simulink library "IOBlock_Library_TTC580"  (R2021a)
settings: Solver=ode45  StartTime=0.0  StopTime=10.0  RelTol=1e-3
PreLoadFcn:
  | addpath(genpath(fileparts(which('IOBlock_Library_TTC580'))));
  | %addpath(genpath(fileparts(which('IOBlock_Library_TTC580.mdl'))))
  | try
  | addpath(genpath([fileparts(which('IOBlock_Library_TTC580')),'\..\DBC_Importer']));
  | addpath(genpath([fileparts(which('IOBlock_Library_TTC580')),'\..\EEPROM_Importer']));
  | addpath(genpath([fileparts(which('IOBlock_Library_TTC580')),'\..\UserDoc']));
  | catch
  | warning('IOBlock_Library_TTC580: add path to DBC_Importer and EEPROM_Importer manually');
  | end
  | try
  | if exist('..\CustomPackage\scripts\OpenAllPackages.m','file')
  |      run('..\CustomPackage\scripts\OpenAllPackages.m'); %always available, ggf. empty
  | end
  | catch
  | warning('A problem occurred opening automatically the CustomPackage. Please open libraries manually');
  | end
  | try
  | set_param(0,'EditorSmartEditingHotParam','off');
  | catch
  | warning('Simlink preferences for ''Edit key parameter when adding new blocks'' needs to be unchecked manually');
  | end
undefined symbols (not defined in the file or in its folder): ADC_Absolute_10V, ADC_Absolute_32V, ADC_Absolute_5V, ADC_BoardTemp, ADC_ChannelInit, ADC_Current, ADC_Get, ADC_K15_, ADC_Ratiometric_10V, ADC_Ratiometric_5V, ADC_Resistive, ADC_SensorSupply, ADC_UBAT, bit_packing, bit_unpacking, CAN_ConfigMsg, compare2error, compare2FET_PROT_REENABLE, crc32_calc_intern, CRC32_EEPROM_Read, CRC32_EEPROM_Write, DIAG_EnterSafestate, DIAG_Status, DIAG_Status_internal, EEPROM_Mirror, EEPROM_Read, EEPROM_Read_OffsetIn, EEPROM_Read_Raw, EEPROM_Write, EEPROM_Write_OffsetIn, EEPROM_Write_Raw, EnterSafestate, FPU_Handler, Get_DI, Get_DI_VarThreshold, Get_K15_, Get_Pulse_Freq_Curr, Get_Pulse_Freq_Volt, Get_WakeUp, GetDateAndTime, IO_ADC_ResetProtection, IO_Blk_Lib_TTC500, IO_CAN_ReadMsg, IO_CAN_WriteMsg, IO_DI_Get, IO_DI_Init, IO_DI_Init_Var, IO_DO_GetCur, IO_DO_GetVoltage, IO_DO_Init, IO_DO_ResetProtection, IO_DO_Set, IO_Driver_GetSerialNumber, IO_Driver_GetVersionOfDriver, IO_Driver_GetVersionOfFPGA, IO_EEPROM_GetStatus, IO_EEPROM_Init, IO_EEPROM_Read_raw, IO_EEPROM_Write, IO_EEPROM_Write_OffsetIn ... (+73)
libraries: simulink x43
(part 17 of 18)

== system IOBlock_Library_TTC580/EEPROM Blocks TTC580 IOlib/EEPROM_Write/IO_EEPROM_Write ==
  EC_Write_Mirror : Inport
  GetStatus : Inport  Port=2
  IO_EEPROM_Write_s : S-Function  FunctionName=IO_EEPROM_Write_s  Parameters=SampleTime,offset,length  SFunctionDeploymentMode=off  EnableBusSupport=off
  ErrorCode : Outport  VectorParamsAs1DForOutWhenUnconnected=off
  wires:
  IO_EEPROM_Write_s/1 -> ErrorCode/1
  GetStatus/1 -> IO_EEPROM_Write_s/2
  EC_Write_Mirror/1 -> IO_EEPROM_Write_s/1

== system IOBlock_Library_TTC580/EEPROM Blocks TTC580 IOlib/EEPROM_Write/Write_Mirror ==
  b_trigger : Inport
  data : Inport  Port=2
  Write_Mirror_s : S-Function  FunctionName=Write_Mirror_s  Parameters=SampleTime,offset,length  SFunctionDeploymentMode=off  EnableBusSupport=off
  ErrorCode_EEPROM_mirror : Outport  VectorParamsAs1DForOutWhenUnconnected=off
  wires:
  Write_Mirror_s/1 -> ErrorCode_EEPROM_mirror/1
  data/1 -> Write_Mirror_s/2
  b_trigger/1 -> Write_Mirror_s/1

== system IOBlock_Library_TTC580/EEPROM Blocks TTC580 IOlib/EEPROM_Write_OffsetIn/EEPROM_Mirror ==
  EC_EEPROM_Init : Inport
  EEPROM_Mirror_s : S-Function  FunctionName=EEPROM_Mirror_s  Parameters=SampleTime,offset,length  SFunctionDeploymentMode=off  EnableBusSupport=off
  Terminator : Terminator
  wires:
  EEPROM_Mirror_s/1 -> Terminator/1
  EC_EEPROM_Init/1 -> EEPROM_Mirror_s/1

== system IOBlock_Library_TTC580/EEPROM Blocks TTC580 IOlib/EEPROM_Write_OffsetIn/IO_EEPROM_GetStatus ==
  IO_EEPROM_GetStatus_s : S-Function  FunctionName=IO_EEPROM_GetStatus_s  Parameters=SampleTime  SFunctionDeploymentMode=off  EnableBusSupport=off
  ErrorCode : Outport  VectorParamsAs1DForOutWhenUnconnected=off
  wires:
  IO_EEPROM_GetStatus_s/1 -> ErrorCode/1

== system IOBlock_Library_TTC580/EEPROM Blocks TTC580 IOlib/EEPROM_Write_OffsetIn/IO_EEPROM_GetStatus1 ==
  IO_EEPROM_GetStatus_s : S-Function  FunctionName=IO_EEPROM_GetStatus_s  Parameters=SampleTime  SFunctionDeploymentMode=off  EnableBusSupport=off
  ErrorCode : Outport  VectorParamsAs1DForOutWhenUnconnected=off
  wires:
  IO_EEPROM_GetStatus_s/1 -> ErrorCode/1

== system IOBlock_Library_TTC580/EEPROM Blocks TTC580 IOlib/EEPROM_Write_OffsetIn/IO_EEPROM_Init ==
  IO_EEPROM_Init_s : S-Function  FunctionName=IO_EEPROM_Init_s  Parameters=SampleTime  SFunctionDeploymentMode=off  EnableBusSupport=off
  ErrorCode : Outport  VectorParamsAs1DForOutWhenUnconnected=off
  wires:
  IO_EEPROM_Init_s/1 -> ErrorCode/1

== system IOBlock_Library_TTC580/EEPROM Blocks TTC580 IOlib/EEPROM_Write_OffsetIn/IO_EEPROM_Write_OffsetIn ==
  offset : Inport
  EC_Write_Mirror : Inport  Port=2
  GetStatus : Inport  Port=3
  IO_EEPROM_Write_OffsetIn_s : S-Function  FunctionName=IO_EEPROM_Write_OffsetIn_s  Parameters=SampleTime,length  SFunctionDeploymentMode=off  EnableBusSupport=off
  ErrorCode : Outport  VectorParamsAs1DForOutWhenUnconnected=off
  wires:
  IO_EEPROM_Write_OffsetIn_s/1 -> ErrorCode/1
  GetStatus/1 -> IO_EEPROM_Write_OffsetIn_s/3
  EC_Write_Mirror/1 -> IO_EEPROM_Write_OffsetIn_s/2
  offset/1 -> IO_EEPROM_Write_OffsetIn_s/1

== system IOBlock_Library_TTC580/EEPROM Blocks TTC580 IOlib/EEPROM_Write_OffsetIn/Write_Mirror_OffsetIn ==
  offset : Inport
  b_trigger : Inport  Port=2
  data : Inport  Port=3
  Write_Mirror_OffsetIn_s : S-Function  FunctionName=Write_Mirror_OffsetIn_s  Parameters=SampleTime,length  SFunctionDeploymentMode=off  EnableBusSupport=off
  ErrorCode_EEPROM_mirror : Outport  VectorParamsAs1DForOutWhenUnconnected=off
  wires:
  Write_Mirror_OffsetIn_s/1 -> ErrorCode_EEPROM_mirror/1
  data/1 -> Write_Mirror_OffsetIn_s/3
  b_trigger/1 -> Write_Mirror_OffsetIn_s/2
  offset/1 -> Write_Mirror_OffsetIn_s/1

== system IOBlock_Library_TTC580/EEPROM Blocks TTC580 IOlib/EEPROM_Write_Raw/IO_EEPROM_Init ==
  IO_EEPROM_Init_s : S-Function  FunctionName=IO_EEPROM_Init_s  Parameters=SampleTime  SFunctionDeploymentMode=off  EnableBusSupport=off
  ErrorCode : Outport  VectorParamsAs1DForOutWhenUnconnected=off
  wires:
  IO_EEPROM_Init_s/1 -> ErrorCode/1

== system IOBlock_Library_TTC580/EEPROM Blocks TTC580 IOlib/EEPROM_Write_Raw/IO_EEPROM_Write_raw ==
  data : Inport
  IO_EEPROM_Write_raw_s : S-Function  FunctionName=IO_EEPROM_Write_raw_s  Parameters=SampleTime,offset,length  SFunctionDeploymentMode=off  EnableBusSupport=off
  ErrorCode : Outport  VectorParamsAs1DForOutWhenUnconnected=off
  wires:
  IO_EEPROM_Write_raw_s/1 -> ErrorCode/1
  data/1 -> IO_EEPROM_Write_raw_s/1

== system IOBlock_Library_TTC580/LIN TTC580 IOlib/IO_LIN_Init/IO_LIN_Init ==
  baudrate : Inport
  checksum_type : Inport  Port=2
  IO_LIN_Init_s : S-Function  FunctionName=IO_LIN_Init_s  Parameters=SampleTime  SFunctionDeploymentMode=off  EnableBusSupport=off
  ErrorCode : Outport  VectorParamsAs1DForOutWhenUnconnected=off
  wires:
  IO_LIN_Init_s/1 -> ErrorCode/1
  checksum_type/1 -> IO_LIN_Init_s/2
  baudrate/1 -> IO_LIN_Init_s/1

== system IOBlock_Library_TTC580/LIN TTC580 IOlib/LIN_Read/LIN_Read_intern ==
  frame_id : Inport
  frame_length : Inport  Port=2
  b_reqst : Inport  Port=3
  LIN_Read_intern_s : S-Function  FunctionName=LIN_Read_intern_s  Parameters=SampleTime  SFunctionDeploymentMode=off  EnableBusSupport=off
  ErrorCode : Outport  VectorParamsAs1DForOutWhenUnconnected=off
  frame_data : Outport  Port=2  VectorParamsAs1DForOutWhenUnconnected=off
  wires:
  LIN_Read_intern_s/2 -> frame_data/1
  LIN_Read_intern_s/1 -> ErrorCode/1
  b_reqst/1 -> LIN_Read_intern_s/3
  frame_length/1 -> LIN_Read_intern_s/2
  frame_id/1 -> LIN_Read_intern_s/1

== system IOBlock_Library_TTC580/LIN TTC580 IOlib/LIN_Write/IO_LIN_Write ==
  frame_id : Inport
  frame_length : Inport  Port=2
  frame_data : Inport  Port=3
  Enable : EnablePort
  IO_LIN_Write_s : S-Function  FunctionName=IO_LIN_Write_s  Parameters=SampleTime  SFunctionDeploymentMode=off  EnableBusSupport=off
  ErrorCode : Outport  VectorParamsAs1DForOutWhenUnconnected=off
  wires:
  IO_LIN_Write_s/1 -> ErrorCode/1
  frame_data/1 -> IO_LIN_Write_s/3
  frame_length/1 -> IO_LIN_Write_s/2
  frame_id/1 -> IO_LIN_Write_s/1

== system IOBlock_Library_TTC580/PVG and VOUT TTC580 IOlib/Set_PVG_Simple/IO_PVG_Init ==
  IO_PVG_Init_s : S-Function  FunctionName=IO_PVG_Init_s  Parameters=SampleTime,pvg_channel,init_output_value  SFunctionDeploymentMode=off  EnableBusSupport=off
  ErrorCode : Outport  VectorParamsAs1DForOutWhenUnconnected=off
  wires:
  IO_PVG_Init_s/1 -> ErrorCode/1

== system IOBlock_Library_TTC580/PVG and VOUT TTC580 IOlib/Set_PVG_Simple/IO_PVG_ResetProtection ==
  Trigger : TriggerPort  VariantControl=(inherit)
  IO_PVG_ResetProtection_s : S-Function  FunctionName=IO_PVG_ResetProtection_s  Parameters=SampleTime,pvg_channel  SFunctionDeploymentMode=off  EnableBusSupport=off
  ErrorCode : Outport  VectorParamsAs1DForOutWhenUnconnected=off
  reset_cnt : Outport  Port=2  VectorParamsAs1DForOutWhenUnconnected=off
  wires:
  IO_PVG_ResetProtection_s/2 -> reset_cnt/1
  IO_PVG_ResetProtection_s/1 -> ErrorCode/1

== system IOBlock_Library_TTC580/PVG and VOUT TTC580 IOlib/Set_PVG_Simple/IO_PVG_SetOutput ==
  output_value : Inport
  IO_PVG_SetOutput_s : S-Function  FunctionName=IO_PVG_SetOutput_s  Parameters=SampleTime,pvg_channel  SFunctionDeploymentMode=off  EnableBusSupport=off
  ErrorCode : Outport  VectorParamsAs1DForOutWhenUnconnected=off
  wires:
  IO_PVG_SetOutput_s/1 -> ErrorCode/1
  output_value/1 -> IO_PVG_SetOutput_s/1

== system IOBlock_Library_TTC580/PVG and VOUT TTC580 IOlib/Set_PVG_Simple/compare2FET_PROT_REENABLE ==
  Errorcode : Inport  OutDataTypeStr=uint16
  compare2error_s : S-Function  FunctionName=compare2error_s  Parameters=SampleTime,define  SFunctionDeploymentMode=off  EnableBusSupport=off
  b_compare : Outport  VectorParamsAs1DForOutWhenUnconnected=off
  wires:
  compare2error_s/1 -> b_compare/1
  Errorcode/1 -> compare2error_s/1

== system IOBlock_Library_TTC580/PVG and VOUT TTC580 IOlib/Set_PVG_VoltFb/IO_PVG_GetVoltage ==
  IO_PVG_GetVoltage_s : S-Function  FunctionName=IO_PVG_GetVoltage_s  Parameters=SampleTime,pvg_channel  SFunctionDeploymentMode=off  EnableBusSupport=off
  ErrorCode : Outport  VectorParamsAs1DForOutWhenUnconnected=off
  voltage : Outport  Port=2  VectorParamsAs1DForOutWhenUnconnected=off
  fresh : Outport  Port=3  VectorParamsAs1DForOutWhenUnconnected=off
  wires:
  IO_PVG_GetVoltage_s/3 -> fresh/1
  IO_PVG_GetVoltage_s/2 -> voltage/1
  IO_PVG_GetVoltage_s/1 -> ErrorCode/1

== system IOBlock_Library_TTC580/PVG and VOUT TTC580 IOlib/Set_PVG_VoltFb/IO_PVG_Init ==
  IO_PVG_Init_s : S-Function  FunctionName=IO_PVG_Init_s  Parameters=SampleTime,pvg_channel,init_output_value  SFunctionDeploymentMode=off  EnableBusSupport=off
  ErrorCode : Outport  VectorParamsAs1DForOutWhenUnconnected=off
  wires:
  IO_PVG_Init_s/1 -> ErrorCode/1

== system IOBlock_Library_TTC580/PVG and VOUT TTC580 IOlib/Set_PVG_VoltFb/IO_PVG_ResetProtection ==
  Trigger : TriggerPort  VariantControl=(inherit)
  IO_PVG_ResetProtection_s : S-Function  FunctionName=IO_PVG_ResetProtection_s  Parameters=SampleTime,pvg_channel  SFunctionDeploymentMode=off  EnableBusSupport=off
  ErrorCode : Outport  VectorParamsAs1DForOutWhenUnconnected=off
  reset_cnt : Outport  Port=2  VectorParamsAs1DForOutWhenUnconnected=off
  wires:
  IO_PVG_ResetProtection_s/1 -> ErrorCode/1
  IO_PVG_ResetProtection_s/2 -> reset_cnt/1

== system IOBlock_Library_TTC580/PVG and VOUT TTC580 IOlib/Set_PVG_VoltFb/IO_PVG_SetOutput ==
  output_value : Inport
  IO_PVG_SetOutput_s : S-Function  FunctionName=IO_PVG_SetOutput_s  Parameters=SampleTime,pvg_channel  SFunctionDeploymentMode=off  EnableBusSupport=off
  ErrorCode : Outport  VectorParamsAs1DForOutWhenUnconnected=off
  wires:
  output_value/1 -> IO_PVG_SetOutput_s/1
  IO_PVG_SetOutput_s/1 -> ErrorCode/1

== system IOBlock_Library_TTC580/PVG and VOUT TTC580 IOlib/Set_PVG_VoltFb/compare2FET_PROT_REENABLE ==
  Errorcode : Inport  OutDataTypeStr=uint16
  compare2error_s : S-Function  FunctionName=compare2error_s  Parameters=SampleTime,define  SFunctionDeploymentMode=off  EnableBusSupport=off
  b_compare : Outport  VectorParamsAs1DForOutWhenUnconnected=off
  wires:
  Errorcode/1 -> compare2error_s/1
  compare2error_s/1 -> b_compare/1

== system IOBlock_Library_TTC580/PVG and VOUT TTC580 IOlib/Set_VOUT_Simple/IO_VOUT_Init ==
  IO_VOUT_Init_s : S-Function  FunctionName=IO_VOUT_Init_s  Parameters=SampleTime,vout_channel  SFunctionDeploymentMode=off  EnableBusSupport=off
  ErrorCode : Outport  VectorParamsAs1DForOutWhenUnconnected=off
  wires:
  IO_VOUT_Init_s/1 -> ErrorCode/1

== system IOBlock_Library_TTC580/PVG and VOUT TTC580 IOlib/Set_VOUT_Simple/IO_VOUT_ResetProtection ==
  Trigger : TriggerPort  VariantControl=(inherit)
  IO_VOUT_ResetProtection_s : S-Function  FunctionName=IO_VOUT_ResetProtection_s  Parameters=SampleTime,vout_channel  SFunctionDeploymentMode=off  EnableBusSupport=off
  ErrorCode : Outport  VectorParamsAs1DForOutWhenUnconnected=off
  reset_cnt : Outport  Port=2  VectorParamsAs1DForOutWhenUnconnected=off
  wires:
  IO_VOUT_ResetProtection_s/2 -> reset_cnt/1
  IO_VOUT_ResetProtection_s/1 -> ErrorCode/1

== system IOBlock_Library_TTC580/PVG and VOUT TTC580 IOlib/Set_VOUT_Simple/IO_VOUT_SetVoltage ==
  output_voltage : Inport
  IO_VOUT_SetVoltage_s : S-Function  FunctionName=IO_VOUT_SetVoltage_s  Parameters=SampleTime,vout_channel  SFunctionDeploymentMode=off  EnableBusSupport=off
  ErrorCode : Outport  VectorParamsAs1DForOutWhenUnconnected=off
  wires:
  IO_VOUT_SetVoltage_s/1 -> ErrorCode/1
  output_voltage/1 -> IO_VOUT_SetVoltage_s/1

== system IOBlock_Library_TTC580/PVG and VOUT TTC580 IOlib/Set_VOUT_Simple/compare2FET_PROT_REENABLE ==
  Errorcode : Inport  OutDataTypeStr=uint16
  compare2error_s : S-Function  FunctionName=compare2error_s  Parameters=SampleTime,define  SFunctionDeploymentMode=off  EnableBusSupport=off
  b_compare : Outport  VectorParamsAs1DForOutWhenUnconnected=off
  wires:
  Errorcode/1 -> compare2error_s/1
  compare2error_s/1 -> b_compare/1

== system IOBlock_Library_TTC580/PVG and VOUT TTC580 IOlib/Set_VOUT_VoltFb/IO_VOUT_GetVoltage ==
  IO_VOUT_GetVoltage_s : S-Function  FunctionName=IO_VOUT_GetVoltage_s  Parameters=SampleTime,vout_channel  SFunctionDeploymentMode=off  EnableBusSupport=off
  ErrorCode : Outport  VectorParamsAs1DForOutWhenUnconnected=off
  voltage : Outport  Port=2  VectorParamsAs1DForOutWhenUnconnected=off
  fresh : Outport  Port=3  VectorParamsAs1DForOutWhenUnconnected=off
  wires:
  IO_VOUT_GetVoltage_s/3 -> fresh/1
  IO_VOUT_GetVoltage_s/2 -> voltage/1
  IO_VOUT_GetVoltage_s/1 -> ErrorCode/1

== system IOBlock_Library_TTC580/PVG and VOUT TTC580 IOlib/Set_VOUT_VoltFb/IO_VOUT_Init ==
  IO_VOUT_Init_s : S-Function  FunctionName=IO_VOUT_Init_s  Parameters=SampleTime,vout_channel  SFunctionDeploymentMode=off  EnableBusSupport=off
  ErrorCode : Outport  VectorParamsAs1DForOutWhenUnconnected=off
  wires:
  IO_VOUT_Init_s/1 -> ErrorCode/1

== system IOBlock_Library_TTC580/PVG and VOUT TTC580 IOlib/Set_VOUT_VoltFb/IO_VOUT_ResetProtection ==
  Trigger : TriggerPort  VariantControl=(inherit)
  IO_VOUT_ResetProtection_s : S-Function  FunctionName=IO_VOUT_ResetProtection_s  Parameters=SampleTime,vout_channel  SFunctionDeploymentMode=off  EnableBusSupport=off
  ErrorCode : Outport  VectorParamsAs1DForOutWhenUnconnected=off
  reset_cnt : Outport  Port=2  VectorParamsAs1DForOutWhenUnconnected=off
  wires:
  IO_VOUT_ResetProtection_s/1 -> ErrorCode/1
  IO_VOUT_ResetProtection_s/2 -> reset_cnt/1

== system IOBlock_Library_TTC580/PVG and VOUT TTC580 IOlib/Set_VOUT_VoltFb/IO_VOUT_SetVoltage ==
  output_voltage : Inport
  IO_VOUT_SetVoltage_s : S-Function  FunctionName=IO_VOUT_SetVoltage_s  Parameters=SampleTime,vout_channel  SFunctionDeploymentMode=off  EnableBusSupport=off
  ErrorCode : Outport  VectorParamsAs1DForOutWhenUnconnected=off
  wires:
  output_voltage/1 -> IO_VOUT_SetVoltage_s/1
  IO_VOUT_SetVoltage_s/1 -> ErrorCode/1

== system IOBlock_Library_TTC580/PVG and VOUT TTC580 IOlib/Set_VOUT_VoltFb/compare2FET_PROT_REENABLE ==
  Errorcode : Inport  OutDataTypeStr=uint16
  compare2error_s : S-Function  FunctionName=compare2error_s  Parameters=SampleTime,define  SFunctionDeploymentMode=off  EnableBusSupport=off
  b_compare : Outport  VectorParamsAs1DForOutWhenUnconnected=off
  wires:
  compare2error_s/1 -> b_compare/1
  Errorcode/1 -> compare2error_s/1

== system IOBlock_Library_TTC580/PWD Blocks TTC580 IOlib/Get_Pulse_Freq_Curr/IO_PWD_ComplexGet ==
  IO_PWD_ComplexGet_s : S-Function  FunctionName=IO_PWD_ComplexGet_s  Parameters=SampleTime,timer_channel,pin_value,pulse_samples  SFunctionDeploymentMode=off  EnableBusSupport=off
  ErrorCode : Outport  VectorParamsAs1DForOutWhenUnconnected=off
  frequency : Outport  Port=2  VectorParamsAs1DForOutWhenUnconnected=off
  pulse_width : Outport  Port=3  VectorParamsAs1DForOutWhenUnconnected=off
  wires:
  IO_PWD_ComplexGet_s/3 -> pulse_width/1
  IO_PWD_ComplexGet_s/2 -> frequency/1
  IO_PWD_ComplexGet_s/1 -> ErrorCode/1

== system IOBlock_Library_TTC580/PWD Blocks TTC580 IOlib/Get_Pulse_Freq_Curr/IO_PWD_ResetProtection ==
  Trigger : TriggerPort  VariantControl=(inherit)
  IO_PWD_ResetProtection_s : S-Function  FunctionName=IO_PWD_ResetProtection_s  Parameters=SampleTime,pwd_channel  SFunctionDeploymentMode=off  EnableBusSupport=off
  ErrorCode : Outport  VectorParamsAs1DForOutWhenUnconnected=off
  reset_cnt : Outport  Port=2  VectorParamsAs1DForOutWhenUnconnected=off
  wires:
  IO_PWD_ResetProtection_s/2 -> reset_cnt/1
  IO_PWD_ResetProtection_s/1 -> ErrorCode/1

== system IOBlock_Library_TTC580/PWD Blocks TTC580 IOlib/Get_Pulse_Freq_Curr/PWD_ComplexInit ==
  PWD_ComplexInit_s : S-Function  FunctionName=PWD_ComplexInit_s  Parameters=SampleTime,timer_channel,pulse_mode,freq_mode,capture_count,pupd,safety_conf  SFunctionDeploymentMode=off  EnableBusSupport=off
  ErrorCode : Outport  VectorParamsAs1DForOutWhenUnconnected=off
  wires:
  PWD_ComplexInit_s/1 -> ErrorCode/1

== system IOBlock_Library_TTC580/PWD Blocks TTC580 IOlib/Get_Pulse_Freq_Curr/compare2FET_PROT_REENABLE ==
  Errorcode : Inport  OutDataTypeStr=uint16
  compare2error_s : S-Function  FunctionName=compare2error_s  Parameters=SampleTime,define  SFunctionDeploymentMode=off  EnableBusSupport=off
  b_compare : Outport  VectorParamsAs1DForOutWhenUnconnected=off
  wires:
  compare2error_s/1 -> b_compare/1
  Errorcode/1 -> compare2error_s/1

== system IOBlock_Library_TTC580/PWD Blocks TTC580 IOlib/Get_Pulse_Freq_Volt/IO_PWD_ComplexGet ==
  IO_PWD_ComplexGet_s : S-Function  FunctionName=IO_PWD_ComplexGet_s  Parameters=SampleTime,timer_channel,pin_value,pulse_samples  SFunctionDeploymentMode=off  EnableBusSupport=off
  ErrorCode : Outport  VectorParamsAs1DForOutWhenUnconnected=off
  frequency : Outport  Port=2  VectorParamsAs1DForOutWhenUnconnected=off
  pulse_width : Outport  Port=3  VectorParamsAs1DForOutWhenUnconnected=off
  wires:
  IO_PWD_ComplexGet_s/1 -> ErrorCode/1
  IO_PWD_ComplexGet_s/2 -> frequency/1
  IO_PWD_ComplexGet_s/3 -> pulse_width/1

== system IOBlock_Library_TTC580/PWD Blocks TTC580 IOlib/Get_Pulse_Freq_Volt/PWD_ComplexInit ==
  PWD_ComplexInit_s : S-Function  FunctionName=PWD_ComplexInit_s  Parameters=SampleTime,timer_channel,pulse_mode,freq_mode,capture_count,pupd,safety_conf  SFunctionDeploymentMode=off  EnableBusSupport=off
  ErrorCode : Outport  VectorParamsAs1DForOutWhenUnconnected=off
  wires:
  PWD_ComplexInit_s/1 -> ErrorCode/1

== system IOBlock_Library_TTC580/PWD Blocks TTC580 IOlib/PWD_Inc/PWD_IncGet ==
  PWD_IncGet_s : S-Function  FunctionName=PWD_IncGet_s  Parameters=SampleTime,inc_channel,pin_value_0,pin_value_1  SFunctionDeploymentMode=off  EnableBusSupport=off
  ErrorCode : Outport  VectorParamsAs1DForOutWhenUnconnected=off
  count : Outport  Port=2  VectorParamsAs1DForOutWhenUnconnected=off
  wires:
  PWD_IncGet_s/1 -> ErrorCode/1
  PWD_IncGet_s/2 -> count/1

== system IOBlock_Library_TTC580/PWD Blocks TTC580 IOlib/PWD_Inc/PWD_IncInit ==
  PWD_IncInit_s : S-Function  FunctionName=PWD_IncInit_s  Parameters=SampleTime,inc_channel,mode,count_init,pupd,safety_conf  SFunctionDeploymentMode=off  EnableBusSupport=off
  ErrorCode : Outport  VectorParamsAs1DForOutWhenUnconnected=off
  wires:
  PWD_IncInit_s/1 -> ErrorCode/1

== system IOBlock_Library_TTC580/PWD Blocks TTC580 IOlib/PWD_IncReset/PWD_IncSet_Internal ==
  count : Inport
  Trigger : TriggerPort  VariantControl=(inherit)
  PWD_IncSet_Internal_s : S-Function  FunctionName=PWD_IncSet_Internal_s  Parameters=SampleTime,inc_channel  SFunctionDeploymentMode=off  EnableBusSupport=off
  ErrorCode : Outport  VectorParamsAs1DForOutWhenUnconnected=off
  wires:
  count/1 -> PWD_IncSet_Internal_s/1
  PWD_IncSet_Internal_s/1 -> ErrorCode/1

== system IOBlock_Library_TTC580/PWM Blocks TTC580 IOlib/Set_PWM_CurrFb/IO_PWM_GetCur ==
  IO_PWM_GetCur_s : S-Function  FunctionName=IO_PWM_GetCur_s  Parameters=SampleTime,pwm_channel  SFunctionDeploymentMode=off  EnableBusSupport=off
  ErrorCode : Outport  VectorParamsAs1DForOutWhenUnconnected=off
  current : Outport  Port=2  VectorParamsAs1DForOutWhenUnconnected=off
  fresh : Outport  Port=3  VectorParamsAs1DForOutWhenUnconnected=off
  wires:
  IO_PWM_GetCur_s/1 -> ErrorCode/1
  IO_PWM_GetCur_s/2 -> current/1
  IO_PWM_GetCur_s/3 -> fresh/1

== system IOBlock_Library_TTC580/PWM Blocks TTC580 IOlib/Set_PWM_CurrFb/IO_PWM_Init ==
  IO_PWM_Init_s : S-Function  FunctionName=IO_PWM_Init_s  Parameters=SampleTime,pwm_channel,frequency,polarity,diag_margin,safety_conf  SFunctionDeploymentMode=off  EnableBusSupport=off
  ErrorCode : Outport  VectorParamsAs1DForOutWhenUnconnected=off
  wires:
  IO_PWM_Init_s/1 -> ErrorCode/1

== system IOBlock_Library_TTC580/PWM Blocks TTC580 IOlib/Set_PWM_CurrFb/IO_PWM_ResetProtection ==
  Trigger : TriggerPort  VariantControl=(inherit)
  IO_PWM_ResetProtection_s : S-Function  FunctionName=IO_PWM_ResetProtection_s  Parameters=SampleTime,pwm_channel  SFunctionDeploymentMode=off  EnableBusSupport=off
  ErrorCode : Outport  VectorParamsAs1DForOutWhenUnconnected=off
  reset_cnt : Outport  Port=2  VectorParamsAs1DForOutWhenUnconnected=off
  wires:
  IO_PWM_ResetProtection_s/1 -> ErrorCode/1
  IO_PWM_ResetProtection_s/2 -> reset_cnt/1

== system IOBlock_Library_TTC580/PWM Blocks TTC580 IOlib/Set_PWM_CurrFb/PWM_SetDuty_Simple ==
  duty_cycle : Inport
  PWM_SetDuty_Simple_s : S-Function  FunctionName=PWM_SetDuty_Simple_s  Parameters=SampleTime,pwm_channel,high_time_fb,period_fb  SFunctionDeploymentMode=off  EnableBusSupport=off
  ErrorCode : Outport  VectorParamsAs1DForOutWhenUnconnected=off
  wires:
  PWM_SetDuty_Simple_s/1 -> ErrorCode/1
  duty_cycle/1 -> PWM_SetDuty_Simple_s/1

== system IOBlock_Library_TTC580/PWM Blocks TTC580 IOlib/Set_PWM_CurrFb/compare2FET_PROT_REENABLE ==
  Errorcode : Inport  OutDataTypeStr=uint16
  compare2error_s : S-Function  FunctionName=compare2error_s  Parameters=SampleTime,define  SFunctionDeploymentMode=off  EnableBusSupport=off
  b_compare : Outport  VectorParamsAs1DForOutWhenUnconnected=off
  wires:
  Errorcode/1 -> compare2error_s/1
  compare2error_s/1 -> b_compare/1

== system IOBlock_Library_TTC580/PWM Blocks TTC580 IOlib/Set_PWM_FullFb/IO_PWM_GetCur ==
  IO_PWM_GetCur_s : S-Function  FunctionName=IO_PWM_GetCur_s  Parameters=SampleTime,pwm_channel  SFunctionDeploymentMode=off  EnableBusSupport=off
  ErrorCode : Outport  VectorParamsAs1DForOutWhenUnconnected=off
  current : Outport  Port=2  VectorParamsAs1DForOutWhenUnconnected=off
  fresh : Outport  Port=3  VectorParamsAs1DForOutWhenUnconnected=off
  wires:
  IO_PWM_GetCur_s/3 -> fresh/1
  IO_PWM_GetCur_s/2 -> current/1
  IO_PWM_GetCur_s/1 -> ErrorCode/1

== system IOBlock_Library_TTC580/PWM Blocks TTC580 IOlib/Set_PWM_FullFb/IO_PWM_Init ==
  IO_PWM_Init_s : S-Function  FunctionName=IO_PWM_Init_s  Parameters=SampleTime,pwm_channel,frequency,polarity,diag_margin,safety_conf  SFunctionDeploymentMode=off  EnableBusSupport=off
  ErrorCode : Outport  VectorParamsAs1DForOutWhenUnconnected=off
  wires:
  IO_PWM_Init_s/1 -> ErrorCode/1

== system IOBlock_Library_TTC580/PWM Blocks TTC580 IOlib/Set_PWM_FullFb/IO_PWM_ResetProtection ==
  Trigger : TriggerPort  VariantControl=(inherit)
  IO_PWM_ResetProtection_s : S-Function  FunctionName=IO_PWM_ResetProtection_s  Parameters=SampleTime,pwm_channel  SFunctionDeploymentMode=off  EnableBusSupport=off
  ErrorCode : Outport  VectorParamsAs1DForOutWhenUnconnected=off
  reset_cnt : Outport  Port=2  VectorParamsAs1DForOutWhenUnconnected=off
  wires:
  IO_PWM_ResetProtection_s/1 -> ErrorCode/1
  IO_PWM_ResetProtection_s/2 -> reset_cnt/1

== system IOBlock_Library_TTC580/PWM Blocks TTC580 IOlib/Set_PWM_FullFb/IO_PWM_SetDuty ==
  duty_cycle : Inport
  IO_PWM_SetDuty_s : S-Function  FunctionName=IO_PWM_SetDuty_s  Parameters=SampleTime,pwm_channel  SFunctionDeploymentMode=off  EnableBusSupport=off
  ErrorCode : Outport  VectorParamsAs1DForOutWhenUnconnected=off
  high_time_fb : Outport  Port=2  VectorParamsAs1DForOutWhenUnconnected=off
  period_fb : Outport  Port=3  VectorParamsAs1DForOutWhenUnconnected=off
  wires:
  duty_cycle/1 -> IO_PWM_SetDuty_s/1
  IO_PWM_SetDuty_s/1 -> ErrorCode/1
  IO_PWM_SetDuty_s/2 -> high_time_fb/1
  IO_PWM_SetDuty_s/3 -> period_fb/1

== system IOBlock_Library_TTC580/PWM Blocks TTC580 IOlib/Set_PWM_FullFb/compare2FET_PROT_REENABLE ==
  Errorcode : Inport  OutDataTypeStr=uint16
  compare2error_s : S-Function  FunctionName=compare2error_s  Parameters=SampleTime,define  SFunctionDeploymentMode=off  EnableBusSupport=off
  b_compare : Outport  VectorParamsAs1DForOutWhenUnconnected=off
  wires:
  Errorcode/1 -> compare2error_s/1
  compare2error_s/1 -> b_compare/1

== system IOBlock_Library_TTC580/PWM Blocks TTC580 IOlib/Set_PWM_Simple/IO_PWM_Init ==
  IO_PWM_Init_s : S-Function  FunctionName=IO_PWM_Init_s  Parameters=SampleTime,pwm_channel,frequency,polarity,diag_margin,safety_conf  SFunctionDeploymentMode=off  EnableBusSupport=off
  ErrorCode : Outport  VectorParamsAs1DForOutWhenUnconnected=off
  wires:
  IO_PWM_Init_s/1 -> ErrorCode/1

== system IOBlock_Library_TTC580/PWM Blocks TTC580 IOlib/Set_PWM_Simple/IO_PWM_ResetProtection ==
  Trigger : TriggerPort  VariantControl=(inherit)
  IO_PWM_ResetProtection_s : S-Function  FunctionName=IO_PWM_ResetProtection_s  Parameters=SampleTime,pwm_channel  SFunctionDeploymentMode=off  EnableBusSupport=off
  ErrorCode : Outport  VectorParamsAs1DForOutWhenUnconnected=off
  reset_cnt : Outport  Port=2  VectorParamsAs1DForOutWhenUnconnected=off
  wires:
  IO_PWM_ResetProtection_s/2 -> reset_cnt/1
  IO_PWM_ResetProtection_s/1 -> ErrorCode/1

== system IOBlock_Library_TTC580/PWM Blocks TTC580 IOlib/Set_PWM_Simple/PWM_SetDuty_Simple ==
  duty_cycle : Inport
  PWM_SetDuty_Simple_s : S-Function  FunctionName=PWM_SetDuty_Simple_s  Parameters=SampleTime,pwm_channel,high_time_fb,period_fb  SFunctionDeploymentMode=off  EnableBusSupport=off
  ErrorCode : Outport  VectorParamsAs1DForOutWhenUnconnected=off
  wires:
  PWM_SetDuty_Simple_s/1 -> ErrorCode/1
  duty_cycle/1 -> PWM_SetDuty_Simple_s/1

== system IOBlock_Library_TTC580/PWM Blocks TTC580 IOlib/Set_PWM_Simple/compare2FET_PROT_REENABLE ==
  Errorcode : Inport  OutDataTypeStr=uint16
  compare2error_s : S-Function  FunctionName=compare2error_s  Parameters=SampleTime,define  SFunctionDeploymentMode=off  EnableBusSupport=off
  b_compare : Outport  VectorParamsAs1DForOutWhenUnconnected=off
  wires:
  Errorcode/1 -> compare2error_s/1
  compare2error_s/1 -> b_compare/1

== system IOBlock_Library_TTC580/SensorSupply TTC580 IOlib/SensorSupply_5V/POWER_Set_Output ==
  mode : Inport
  POWER_Set_Output_s : S-Function  FunctionName=POWER_Set_Output_s  Parameters=SampleTime,pin  SFunctionDeploymentMode=off  EnableBusSupport=off
  ErrorCode : Outport  VectorParamsAs1DForOutWhenUnconnected=off
  wires:
  mode/1 -> POWER_Set_Output_s/1
  POWER_Set_Output_s/1 -> ErrorCode/1

== system IOBlock_Library_TTC580/SensorSupply TTC580 IOlib/SensorSupply_Modif/POWER_Set_Output ==
  mode : Inport
  POWER_Set_Output_s : S-Function  FunctionName=POWER_Set_Output_s  Parameters=SampleTime,pin  SFunctionDeploymentMode=off  EnableBusSupport=off
  ErrorCode : Outport  VectorParamsAs1DForOutWhenUnconnected=off
  wires:
  POWER_Set_Output_s/1 -> ErrorCode/1
  mode/1 -> POWER_Set_Output_s/1

== system IOBlock_Library_TTC580/System  Blocks TTC580 IOlib/DIAG_Status/Compare To Constant ==
  FPGA_Major : Inport
  Constant : Constant  Value=FPGA_Major  OutDataTypeStr=Inherit: Inherit via back propagation
  Relational Operator : RelationalOperator  Operator===  OutDataTypeStr=boolean  RndMeth=Simplest
  y : Outport  VectorParamsAs1DForOutWhenUnconnected=off
  wires:
  Relational Operator/1 -> y/1
  Constant/1 -> Relational Operator/2
  FPGA_Major/1 -> Relational Operator/1

== system IOBlock_Library_TTC580/System  Blocks TTC580 IOlib/DIAG_Status/Compare To Constant1 ==
  FPGA_Minor : Inport
  Constant : Constant  Value=FPGA_Minor  OutDataTypeStr=Inherit: Inherit via back propagation
  Relational Operator : RelationalOperator  Operator===  OutDataTypeStr=boolean  RndMeth=Simplest
  y : Outport  VectorParamsAs1DForOutWhenUnconnected=off
  wires:
  FPGA_Minor/1 -> Relational Operator/1
  Constant/1 -> Relational Operator/2
  Relational Operator/1 -> y/1

== system IOBlock_Library_TTC580/System  Blocks TTC580 IOlib/DIAG_Status/Compare To Constant2 ==
  IODriver_Major : Inport
  Constant : Constant  Value=IODriver_Major  OutDataTypeStr=Inherit: Inherit via back propagation
  Relational Operator : RelationalOperator  Operator===  OutDataTypeStr=boolean  RndMeth=Simplest
  y : Outport  VectorParamsAs1DForOutWhenUnconnected=off
  wires:
  Relational Operator/1 -> y/1
  Constant/1 -> Relational Operator/2
  IODriver_Major/1 -> Relational Operator/1

== system IOBlock_Library_TTC580/System  Blocks TTC580 IOlib/DIAG_Status/Compare To Constant3 ==
  IODriver_Minor : Inport
  Constant : Constant  Value=IODriver_Minor  OutDataTypeStr=Inherit: Inherit via back propagation
  Relational Operator : RelationalOperator  Operator===  OutDataTypeStr=boolean  RndMeth=Simplest
  y : Outport  VectorParamsAs1DForOutWhenUnconnected=off
  wires:
  IODriver_Minor/1 -> Relational Operator/1
  Constant/1 -> Relational Operator/2
  Relational Operator/1 -> y/1

== system IOBlock_Library_TTC580/System  Blocks TTC580 IOlib/DIAG_Status/DIAG_Status_internal ==
  DIAG_Status_internal_s : S-Function  FunctionName=DIAG_Status_internal_s  Parameters=SampleTime  SFunctionDeploymentMode=off  EnableBusSupport=off
  ErrorCode : Outport  VectorParamsAs1DForOutWhenUnconnected=off
  diag_state : Outport  Port=2  VectorParamsAs1DForOutWhenUnconnected=off
  watchdog_state : Outport  Port=3  VectorParamsAs1DForOutWhenUnconnected=off
  diag_error_error_code : Outport  Port=4  VectorParamsAs1DForOutWhenUnconnected=off
  diag_error_device_num : Outport  Port=5  VectorParamsAs1DForOutWhenUnconnected=off
  diag_error_faulty_value : Outport  Port=6  VectorParamsAs1DForOutWhenUnconnected=off
  watchdog_error_error_code : Outport  Port=7  VectorParamsAs1DForOutWhenUnconnected=off
  watchdog_error_device_num : Outport  Port=8  VectorParamsAs1DForOutWhenUnconnected=off
  watchdog_error_faulty_value : Outport  Port=9  VectorParamsAs1DForOutWhenUnconnected=off
  error_count : Outport  Port=10  VectorParamsAs1DForOutWhenUnconnected=off
  wires:
  DIAG_Status_internal_s/1 -> ErrorCode/1
  DIAG_Status_internal_s/2 -> diag_state/1
  DIAG_Status_internal_s/3 -> watchdog_state/1
  DIAG_Status_internal_s/4 -> diag_error_error_code/1
  DIAG_Status_internal_s/5 -> diag_error_device_num/1
  DIAG_Status_internal_s/6 -> diag_error_faulty_value/1
  DIAG_Status_internal_s/7 -> watchdog_error_error_code/1
  DIAG_Status_internal_s/8 -> watchdog_error_device_num/1
  DIAG_Status_internal_s/9 -> watchdog_error_faulty_value/1
  DIAG_Status_internal_s/10 -> error_count/1

== system IOBlock_Library_TTC580/System  Blocks TTC580 IOlib/DIAG_Status/IO_Driver_GetVersionOfDriver ==
  IO_Driver_GetVersionOfDriver_s : S-Function  FunctionName=IO_Driver_GetVersionOfDriver_s  Parameters=SampleTime  SFunctionDeploymentMode=off  EnableBusSupport=off
  ErrorCode : Outport  VectorParamsAs1DForOutWhenUnconnected=off
  major : Outport  Port=2  VectorParamsAs1DForOutWhenUnconnected=off
  minor : Outport  Port=3  VectorParamsAs1DForOutWhenUnconnected=off
  patchlevel : Outport  Port=4  VectorParamsAs1DForOutWhenUnconnected=off
  wires:
  IO_Driver_GetVersionOfDriver_s/1 -> ErrorCode/1
  IO_Driver_GetVersionOfDriver_s/2 -> major/1
  IO_Driver_GetVersionOfDriver_s/3 -> minor/1
  IO_Driver_GetVersionOfDriver_s/4 -> patchlevel/1

== system IOBlock_Library_TTC580/System  Blocks TTC580 IOlib/DIAG_Status/IO_Driver_GetVersionOfFPGA ==
  IO_Driver_GetVersionOfFPGA_s : S-Function  FunctionName=IO_Driver_GetVersionOfFPGA_s  Parameters=SampleTime  SFunctionDeploymentMode=off  EnableBusSupport=off
  ErrorCode : Outport  VectorParamsAs1DForOutWhenUnconnected=off
  rev0 : Outport  Port=2  VectorParamsAs1DForOutWhenUnconnected=off
  rev1 : Outport  Port=3  VectorParamsAs1DForOutWhenUnconnected=off
  rev2 : Outport  Port=4  VectorParamsAs1DForOutWhenUnconnected=off
  device : Outport  Port=5  VectorParamsAs1DForOutWhenUnconnected=off
  release : Outport  Port=6  VectorParamsAs1DForOutWhenUnconnected=off
  patchlevel : Outport  Port=7  VectorParamsAs1DForOutWhenUnconnected=off
  wires:
  IO_Driver_GetVersionOfFPGA_s/1 -> ErrorCode/1
  IO_Driver_GetVersionOfFPGA_s/2 -> rev0/1
  IO_Driver_GetVersionOfFPGA_s/3 -> rev1/1
  IO_Driver_GetVersionOfFPGA_s/4 -> rev2/1
  IO_Driver_GetVersionOfFPGA_s/5 -> device/1
  IO_Driver_GetVersionOfFPGA_s/6 -> release/1
  IO_Driver_GetVersionOfFPGA_s/7 -> patchlevel/1

== system IOBlock_Library_TTC580/System  Blocks TTC580 IOlib/EnterSafestate/DIAG_EnterSafestate_x ==
  Enable : EnablePort
  DIAG_EnterSafestate_s : S-Function  FunctionName=DIAG_EnterSafestate_s  Parameters=SampleTime  SFunctionDeploymentMode=off  EnableBusSupport=off
  ErrorCode : Outport  VectorParamsAs1DForOutWhenUnconnected=off
  wires:
  DIAG_EnterSafestate_s/1 -> ErrorCode/1

== system IOBlock_Library_TTC580/System  Blocks TTC580 IOlib/GetDateAndTime/IO_RTC_GetDateAndTime ==
  Trigger : TriggerPort  VariantControl=(inherit)  ZeroCross=off
  IO_RTC_GetDateAndTime_s : S-Function  FunctionName=IO_RTC_GetDateAndTime_s  Parameters=SampleTime  SFunctionDeploymentMode=off  EnableBusSupport=off
  ErrorCode : Outport  VectorParamsAs1DForOutWhenUnconnected=off
  seconds : Outport  Port=2  VectorParamsAs1DForOutWhenUnconnected=off
  minutes : Outport  Port=3  VectorParamsAs1DForOutWhenUnconnected=off
  hours : Outport  Port=4  VectorParamsAs1DForOutWhenUnconnected=off
  days : Outport  Port=5  VectorParamsAs1DForOutWhenUnconnected=off
  months : Outport  Port=6  VectorParamsAs1DForOutWhenUnconnected=off
  years : Outport  Port=7  VectorParamsAs1DForOutWhenUnconnected=off
  wires:
  IO_RTC_GetDateAndTime_s/7 -> years/1
  IO_RTC_GetDateAndTime_s/6 -> months/1
  IO_RTC_GetDateAndTime_s/5 -> days/1
  IO_RTC_GetDateAndTime_s/4 -> hours/1
  IO_RTC_GetDateAndTime_s/3 -> minutes/1
  IO_RTC_GetDateAndTime_s/2 -> seconds/1
  IO_RTC_GetDateAndTime_s/1 -> ErrorCode/1

== system IOBlock_Library_TTC580/System  Blocks TTC580 IOlib/GetDateAndTime/IO_RTC_GetDateAndTimeStatus ==
  logical_link : Inport
  IO_RTC_GetDateAndTimeStatus_s : S-Function  FunctionName=IO_RTC_GetDateAndTimeStatus_s  Parameters=SampleTime  SFunctionDeploymentMode=off  EnableBusSupport=off
  ErrorCode : Outport  VectorParamsAs1DForOutWhenUnconnected=off
  wires:
  logical_link/1 -> IO_RTC_GetDateAndTimeStatus_s/1
  IO_RTC_GetDateAndTimeStatus_s/1 -> ErrorCode/1

== system IOBlock_Library_TTC580/System  Blocks TTC580 IOlib/GetDateAndTime/IO_RTC_InitDateAndTime ==
  IO_RTC_InitDateAndTime_s : S-Function  FunctionName=IO_RTC_InitDateAndTime_s  Parameters=SampleTime  SFunctionDeploymentMode=off  EnableBusSupport=off
  ErrorCode : Outport  VectorParamsAs1DForOutWhenUnconnected=off
  wires:
  IO_RTC_InitDateAndTime_s/1 -> ErrorCode/1

== system IOBlock_Library_TTC580/System  Blocks TTC580 IOlib/MainDlg/MainDlg_basic ==
  MainDlg_basic_s : S-Function  FunctionName=MainDlg_basic_s  Parameters=SampleTime,baudrate_CAN0,tseg1_CAN0,tseg2_CAN0,sjw_CAN0,brp_CAN0,baudrate_CAN1,tseg1_CAN1,tseg2_CAN1,sjw_CAN1,brp_CAN1,baudrate_CAN2,tseg1_CAN2,tseg2_CAN2,sjw_CAN2,brp_CAN2,baudrate_CAN3,baudrate_CAN4,baudrate_CAN5,baudrate_CAN6,tseg1,tseg2,sjw,Duration_ms,glitch_filter_time,watchdog_window_size,watchdog_reset_behavior,brp,Major_Number,Minor_Number,Revison_Number,Node_Number,Enable_Reset_by_TTCDownloader,Enable_CCP,CRO_ID,DTO_ID,CCP_Station_Addr,CCP_Station_ID,CPP_channel,CPP_id_format,bEnable_DAQ0,bEnable_DAQ1_2,ODT_total,bEnable_ErrorCBAction,bDIAG_ERR_DISABLE_SSW0,bDIAG_ERR_DISABLE_SSW1,bDIAG_ERR_DISABLE_SSW2,bFlashOverEthernet  SFunctionDeploymentMode=off  EnableBusSupport=off
  ErrorCode : Outport
  ExecutionTime : Outport  Port=2
  wires:
  MainDlg_basic_s/2 -> ExecutionTime/1
  MainDlg_basic_s/1 -> ErrorCode/1

== system IOBlock_Library_TTC580/System  Blocks TTC580 IOlib/Postrun_Enable/IO_POWER_Get_KL15 ==
  IO_POWER_Get_s : S-Function  FunctionName=IO_POWER_Get_s  Parameters=SampleTime,pin  SFunctionDeploymentMode=off  EnableBusSupport=off
  ErrorCode : Outport  VectorParamsAs1DForOutWhenUnconnected=off
  state : Outport  Port=2  VectorParamsAs1DForOutWhenUnconnected=off
  wires:
  IO_POWER_Get_s/1 -> ErrorCode/1
  IO_POWER_Get_s/2 -> state/1

== system IOBlock_Library_TTC580/System  Blocks TTC580 IOlib/Postrun_Enable/IO_POWER_Set_KL15 ==
  mode : Inport
  IO_POWER_Set_s : S-Function  FunctionName=IO_POWER_Set_s  Parameters=SampleTime,pin  SFunctionDeploymentMode=off  EnableBusSupport=off
  ErrorCode : Outport  VectorParamsAs1DForOutWhenUnconnected=off
  wires:
  mode/1 -> IO_POWER_Set_s/1
  IO_POWER_Set_s/1 -> ErrorCode/1

== system IOBlock_Library_TTC580/System  Blocks TTC580 IOlib/Power_Enable/IO_POWER_Set_POWERSTAGE ==
  mode : Inport
  IO_POWER_Set_s : S-Function  FunctionName=IO_POWER_Set_s  Parameters=SampleTime,pin  SFunctionDeploymentMode=off  EnableBusSupport=off
  ErrorCode : Outport  VectorParamsAs1DForOutWhenUnconnected=off
  wires:
  IO_POWER_Set_s/1 -> ErrorCode/1
  mode/1 -> IO_POWER_Set_s/1

== system IOBlock_Library_TTC580/System  Blocks TTC580 IOlib/Power_Enable/IO_POWER_Set_SSW0 ==
  mode : Inport
  IO_POWER_Set_s : S-Function  FunctionName=IO_POWER_Set_s  Parameters=SampleTime,pin  SFunctionDeploymentMode=off  EnableBusSupport=off
  ErrorCode : Outport  VectorParamsAs1DForOutWhenUnconnected=off
  wires:
  mode/1 -> IO_POWER_Set_s/1
  IO_POWER_Set_s/1 -> ErrorCode/1

== system IOBlock_Library_TTC580/System  Blocks TTC580 IOlib/Power_Enable/IO_POWER_Set_SSW1 ==
  mode : Inport
  IO_POWER_Set_s : S-Function  FunctionName=IO_POWER_Set_s  Parameters=SampleTime,pin  SFunctionDeploymentMode=off  EnableBusSupport=off
  ErrorCode : Outport  VectorParamsAs1DForOutWhenUnconnected=off
  wires:
  mode/1 -> IO_POWER_Set_s/1
  IO_POWER_Set_s/1 -> ErrorCode/1

== system IOBlock_Library_TTC580/System  Blocks TTC580 IOlib/Power_Enable/IO_POWER_Set_SSW2 ==
  mode : Inport
  IO_POWER_Set_s : S-Function  FunctionName=IO_POWER_Set_s  Parameters=SampleTime,pin  SFunctionDeploymentMode=off  EnableBusSupport=off
  ErrorCode : Outport  VectorParamsAs1DForOutWhenUnconnected=off
  wires:
  mode/1 -> IO_POWER_Set_s/1
  IO_POWER_Set_s/1 -> ErrorCode/1

== system IOBlock_Library_TTC580/System  Blocks TTC580 IOlib/SetDateAndTime/IO_RTC_GetDateAndTimeStatus ==
  logical_link : Inport
  IO_RTC_GetDateAndTimeStatus_s : S-Function  FunctionName=IO_RTC_GetDateAndTimeStatus_s  Parameters=SampleTime  SFunctionDeploymentMode=off  EnableBusSupport=off
  ErrorCode : Outport  VectorParamsAs1DForOutWhenUnconnected=off
  wires:
  IO_RTC_GetDateAndTimeStatus_s/1 -> ErrorCode/1
  logical_link/1 -> IO_RTC_GetDateAndTimeStatus_s/1

== system IOBlock_Library_TTC580/System  Blocks TTC580 IOlib/SetDateAndTime/IO_RTC_InitDateAndTime ==
  IO_RTC_InitDateAndTime_s : S-Function  FunctionName=IO_RTC_InitDateAndTime_s  Parameters=SampleTime  SFunctionDeploymentMode=off  EnableBusSupport=off
  ErrorCode : Outport  VectorParamsAs1DForOutWhenUnconnected=off
  wires:
  IO_RTC_InitDateAndTime_s/1 -> ErrorCode/1

== system IOBlock_Library_TTC580/System  Blocks TTC580 IOlib/SetDateAndTime/IO_RTC_SetDateAndTime ==
  seconds : Inport
  minutes : Inport  Port=2
  hours : Inport  Port=3
  days : Inport  Port=4
  months : Inport  Port=5
  years : Inport  Port=6
  Trigger : TriggerPort  VariantControl=(inherit)
  IO_RTC_SetDateAndTime_s : S-Function  FunctionName=IO_RTC_SetDateAndTime_s  Parameters=SampleTime  SFunctionDeploymentMode=off  EnableBusSupport=off
  ErrorCode : Outport  VectorParamsAs1DForOutWhenUnconnected=off
  wires:
  IO_RTC_SetDateAndTime_s/1 -> ErrorCode/1
  years/1 -> IO_RTC_SetDateAndTime_s/6
  months/1 -> IO_RTC_SetDateAndTime_s/5
  days/1 -> IO_RTC_SetDateAndTime_s/4
  hours/1 -> IO_RTC_SetDateAndTime_s/3
  minutes/1 -> IO_RTC_SetDateAndTime_s/2
  seconds/1 -> IO_RTC_SetDateAndTime_s/1

== system IOBlock_Library_TTC580/UART TTC580 IOlib/UART_Read/IO_UART_Init ==
  IO_UART_Init_s : S-Function  FunctionName=IO_UART_Init_s  Parameters=SampleTime,baudrate,dbits,par,sbits  SFunctionDeploymentMode=off  EnableBusSupport=off
  ErrorCode : Outport  VectorParamsAs1DForOutWhenUnconnected=off
  wires:
  IO_UART_Init_s/1 -> ErrorCode/1

== system IOBlock_Library_TTC580/UART TTC580 IOlib/UART_Read/IO_UART_Read ==
  len : Inport
  IO_UART_Read_s : S-Function  FunctionName=IO_UART_Read_s  Parameters=SampleTime  SFunctionDeploymentMode=off  EnableBusSupport=off
  ErrorCode : Outport  VectorParamsAs1DForOutWhenUnconnected=off
  data : Outport  Port=2  VectorParamsAs1DForOutWhenUnconnected=off
  rx_len : Outport  Port=3  VectorParamsAs1DForOutWhenUnconnected=off
  wires:
  len/1 -> IO_UART_Read_s/1
  IO_UART_Read_s/1 -> ErrorCode/1
  IO_UART_Read_s/2 -> data/1
  IO_UART_Read_s/3 -> rx_len/1

== system IOBlock_Library_TTC580/UART TTC580 IOlib/UART_Write/IO_UART_Init ==
  IO_UART_Init_s : S-Function  FunctionName=IO_UART_Init_s  Parameters=SampleTime,baudrate,dbits,par,sbits  SFunctionDeploymentMode=off  EnableBusSupport=off
  ErrorCode : Outport  VectorParamsAs1DForOutWhenUnconnected=off
  wires:
  IO_UART_Init_s/1 -> ErrorCode/1

== system IOBlock_Library_TTC580/UART TTC580 IOlib/UART_Write/IO_UART_Write ==
  data : Inport
  len : Inport  Port=2
  Enable : EnablePort
  IO_UART_Write_s : S-Function  FunctionName=IO_UART_Write_s  Parameters=SampleTime  SFunctionDeploymentMode=off  EnableBusSupport=off
  ErrorCode : Outport  VectorParamsAs1DForOutWhenUnconnected=off
  tx_len : Outport  Port=2  VectorParamsAs1DForOutWhenUnconnected=off
  wires:
  IO_UART_Write_s/2 -> tx_len/1
  IO_UART_Write_s/1 -> ErrorCode/1
  len/1 -> IO_UART_Write_s/2
  data/1 -> IO_UART_Write_s/1

== system IOBlock_Library_TTC580/UART TTC580 IOlib/UART_Write/Trigger ==
  Compare To Constant : simulink/Logic and Bit Operations/Compare To Constant  relop===  const=max(derate - 1,0)  OutDataTypeStr=boolean  ZeroCross=off
  Counter Limited : simulink/Sources/Counter Limited  uplimit=max(derate - 1,0)  tsamp=-1
  Trigger : Outport  VectorParamsAs1DForOutWhenUnconnected=off
  wires:
  Compare To Constant/1 -> Trigger/1
  Counter Limited/1 -> Compare To Constant/1

== system IOBlock_Library_TTC580/UART TTC580 IOlib/UART_Write/snprintf ==
  value : Inport
  snprintf_s : S-Function  FunctionName=snprintf_s  Parameters=SampleTime,max_size,Comment  SFunctionDeploymentMode=off  EnableBusSupport=off
  NumOfChar : Outport  VectorParamsAs1DForOutWhenUnconnected=off
  str_out : Outport  Port=2  VectorParamsAs1DForOutWhenUnconnected=off
  wires:
  snprintf_s/2 -> str_out/1
  snprintf_s/1 -> NumOfChar/1
  value/1 -> snprintf_s/1

== system IOBlock_Library_TTC580/UART TTC580 IOlib/Write_RS232_/IO_UART_Init ==
  IO_UART_Init_s : S-Function  FunctionName=IO_UART_Init_s  Parameters=SampleTime,baudrate,dbits,par,sbits  SFunctionDeploymentMode=off  EnableBusSupport=off
  ErrorCode : Outport  VectorParamsAs1DForOutWhenUnconnected=off
  wires:
  IO_UART_Init_s/1 -> ErrorCode/1

== system IOBlock_Library_TTC580/UART TTC580 IOlib/Write_RS232_/IO_UART_Write ==
  data : Inport
  len : Inport  Port=2
  Enable : EnablePort
  IO_UART_Write_s : S-Function  FunctionName=IO_UART_Write_s  Parameters=SampleTime  SFunctionDeploymentMode=off  EnableBusSupport=off
  ErrorCode : Outport  VectorParamsAs1DForOutWhenUnconnected=off
  tx_len : Outport  Port=2  VectorParamsAs1DForOutWhenUnconnected=off
  wires:
  data/1 -> IO_UART_Write_s/1
  len/1 -> IO_UART_Write_s/2
  IO_UART_Write_s/1 -> ErrorCode/1
  IO_UART_Write_s/2 -> tx_len/1

== system IOBlock_Library_TTC580/UART TTC580 IOlib/Write_RS232_/Trigger ==
  Compare To Constant : simulink/Logic and Bit Operations/Compare To Constant  relop===  const=max(derate - 1,0)  OutDataTypeStr=boolean  ZeroCross=off
  Counter Limited : simulink/Sources/Counter Limited  uplimit=max(derate - 1,0)  tsamp=-1
  Trigger : Outport  VectorParamsAs1DForOutWhenUnconnected=off
  wires:
  Counter Limited/1 -> Compare To Constant/1
  Compare To Constant/1 -> Trigger/1

== system IOBlock_Library_TTC580/UART TTC580 IOlib/Write_RS232_/snprintf_merge_printf ==
  value : Inport
  snprintf_merge_printf_s : S-Function  FunctionName=snprintf_merge_printf_s  Parameters=SampleTime,max_size,Comment  SFunctionDeploymentMode=off  EnableBusSupport=off
  NumOfChar : Outport  VectorParamsAs1DForOutWhenUnconnected=off
  str_out : Outport  Port=2  VectorParamsAs1DForOutWhenUnconnected=off
  wires:
  value/1 -> snprintf_merge_printf_s/1
  snprintf_merge_printf_s/1 -> NumOfChar/1
  snprintf_merge_printf_s/2 -> str_out/1

== system IOBlock_Library_TTC580/UART TTC580 IOlib/Write_RS232_green/IO_UART_Init ==
  IO_UART_Init_s : S-Function  FunctionName=IO_UART_Init_s  Parameters=SampleTime,baudrate,dbits,par,sbits  SFunctionDeploymentMode=off  EnableBusSupport=off
  ErrorCode : Outport  VectorParamsAs1DForOutWhenUnconnected=off
  wires:
  IO_UART_Init_s/1 -> ErrorCode/1

== system IOBlock_Library_TTC580/UART TTC580 IOlib/Write_RS232_green/IO_UART_Write ==
  data : Inport
  len : Inport  Port=2
  Enable : EnablePort
  IO_UART_Write_s : S-Function  FunctionName=IO_UART_Write_s  Parameters=SampleTime  SFunctionDeploymentMode=off  EnableBusSupport=off
  ErrorCode : Outport  VectorParamsAs1DForOutWhenUnconnected=off
  tx_len : Outport  Port=2  VectorParamsAs1DForOutWhenUnconnected=off
  wires:
  data/1 -> IO_UART_Write_s/1
  len/1 -> IO_UART_Write_s/2
  IO_UART_Write_s/1 -> ErrorCode/1
  IO_UART_Write_s/2 -> tx_len/1

== system IOBlock_Library_TTC580/UART TTC580 IOlib/Write_RS232_green/Trigger ==
  Compare To Constant : simulink/Logic and Bit Operations/Compare To Constant  relop===  const=max(derate - 1,0)  OutDataTypeStr=boolean  ZeroCross=off
  Counter Limited : simulink/Sources/Counter Limited  uplimit=max(derate - 1,0)  tsamp=-1
  Trigger : Outport  VectorParamsAs1DForOutWhenUnconnected=off
  wires:
  Counter Limited/1 -> Compare To Constant/1
  Compare To Constant/1 -> Trigger/1

== system IOBlock_Library_TTC580/UART TTC580 IOlib/Write_RS232_green/snprintf_merge_printf ==
  value : Inport
  snprintf_merge_printf_s : S-Function  FunctionName=snprintf_merge_printf_s  Parameters=SampleTime,max_size,Comment  SFunctionDeploymentMode=off  EnableBusSupport=off
  NumOfChar : Outport  VectorParamsAs1DForOutWhenUnconnected=off
  str_out : Outport  Port=2  VectorParamsAs1DForOutWhenUnconnected=off
  wires:
  value/1 -> snprintf_merge_printf_s/1
  snprintf_merge_printf_s/1 -> NumOfChar/1
  snprintf_merge_printf_s/2 -> str_out/1

== system IOBlock_Library_TTC580/UART TTC580 IOlib/Write_RS232_red/IO_UART_Init ==
  IO_UART_Init_s : S-Function  FunctionName=IO_UART_Init_s  Parameters=SampleTime,baudrate,dbits,par,sbits  SFunctionDeploymentMode=off  EnableBusSupport=off
  ErrorCode : Outport  VectorParamsAs1DForOutWhenUnconnected=off
  wires:
  IO_UART_Init_s/1 -> ErrorCode/1

== system IOBlock_Library_TTC580/UART TTC580 IOlib/Write_RS232_red/IO_UART_Write ==
  data : Inport
  len : Inport  Port=2
  Enable : EnablePort
  IO_UART_Write_s : S-Function  FunctionName=IO_UART_Write_s  Parameters=SampleTime  SFunctionDeploymentMode=off  EnableBusSupport=off
  ErrorCode : Outport  VectorParamsAs1DForOutWhenUnconnected=off
  tx_len : Outport  Port=2  VectorParamsAs1DForOutWhenUnconnected=off
  wires:
  data/1 -> IO_UART_Write_s/1
  len/1 -> IO_UART_Write_s/2
  IO_UART_Write_s/1 -> ErrorCode/1
  IO_UART_Write_s/2 -> tx_len/1

== system IOBlock_Library_TTC580/UART TTC580 IOlib/Write_RS232_red/Trigger ==
  Compare To Constant : simulink/Logic and Bit Operations/Compare To Constant  relop===  const=max(derate - 1,0)  OutDataTypeStr=boolean  ZeroCross=off
  Counter Limited : simulink/Sources/Counter Limited  uplimit=max(derate - 1,0)  tsamp=-1
  Trigger : Outport  VectorParamsAs1DForOutWhenUnconnected=off
  wires:
  Counter Limited/1 -> Compare To Constant/1
  Compare To Constant/1 -> Trigger/1

== system IOBlock_Library_TTC580/UART TTC580 IOlib/Write_RS232_red/snprintf_merge_printf ==
  value : Inport
  snprintf_merge_printf_s : S-Function  FunctionName=snprintf_merge_printf_s  Parameters=SampleTime,max_size,Comment  SFunctionDeploymentMode=off  EnableBusSupport=off
  NumOfChar : Outport  VectorParamsAs1DForOutWhenUnconnected=off
  str_out : Outport  Port=2  VectorParamsAs1DForOutWhenUnconnected=off
  wires:
  value/1 -> snprintf_merge_printf_s/1
  snprintf_merge_printf_s/1 -> NumOfChar/1
  snprintf_merge_printf_s/2 -> str_out/1
